simulink model "one_channel"  (R2022b)
settings: Solver=FixedStepAuto  StartTime=0.0  StopTime=3  FixedStep=1/fs  RelTol=1e-3
settings Model: Creator=joaovitor  LastModifiedBy=joaovitor

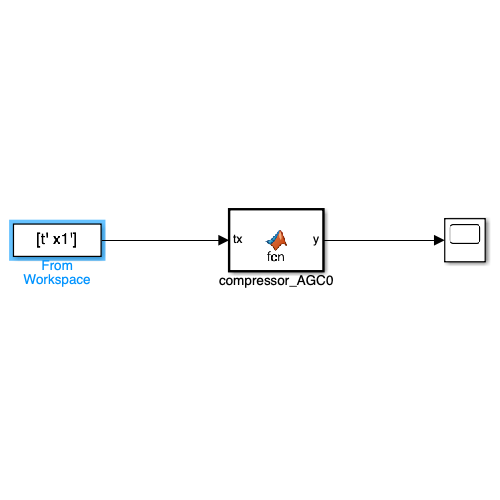
[thumbnail: Simulink's stored preview of the top-level diagram]
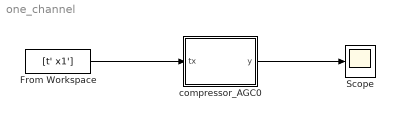
== system one_channel ==
  From Workspace : FromWorkspace  VariableName=[t' x1']
  Scope : Scope
  compressor_AGC0 : MATLAB Function  TreatAsAtomicUnit=on
  wires:
  From Workspace/1 -> compressor_AGC0/1(tx)
  compressor_AGC0/1(y) -> Scope/1

== matlab function one_channel/compressor_AGC0 ==
  data: tx input; y output
function y = fcn(tx)
    % Assume tx is a two-column matrix [t, x]
    
    % Extract the signal part
    x = tx(:, 1);  % Second column contains the signal (x1)

    % Parameters
    threshold = -10;       % Example threshold value (dBFS)
    ratio = 2;             % Compression ratio
    fs = 1000;             % Sampling frequency (Hz)
    attack_time = 0.1;     % Attack time in seconds
    release_time = 0.2;    % Release time in seconds

    % Call the custom compressor function
    y_signal = compressor_AGC(x, threshold, ratio, fs, attack_time, release_time);
    
    % Combine the time vector and compressed signal for output
    y = [tx(:, 1), y_signal]; % Reattach the time vector to the output
end
